simulink model "PTB_BatteryElectricVehicles"  (R2018b)
settings: Solver=ode23tb  StartTime=0.0  StopTime=3158  FixedStep=.001  RelTol=1e-5
model workspace (MAT data in the model file):
  Cd = 0.3
  DrCycles : struct (value not decoded)
  DriveCycleTime = 3158
  MCOS : class17 (value not decoded)
  I = 1
  Kbr = 5000
  P = 200
  axle_b = 10
  axle_k = 0.3
  bevAxle_wc = 400
  bevNp = 1
  bevNs = 8
  diffRatio = 1
  diffRatio1 = 1
  motorMaxTorqueNm = [0.6 0.6 0.8 0.9 2.2 2.9 5.1 7.8 11.3 15.3 20 25 ... (40 elements, 40x1)]
  motorSpeedRadPs = [90.118 90.118 90.118 90.118 90.01333333 89.804 89.49 89.07133333 88.65266667 88.12933333 87.39666667 86.87333333 ... (39 elements, 39x1)]
  vehicleMass = 365
  wheelRadius = 0.3
undefined symbols (not defined in the file): Driver, Wheels_Driver_VehDyn_Lib
libraries: autolibshared x3, simulink x2, autolibdatasheetbattery x1, autolibmappedmotor x1
(part 3 of 3)

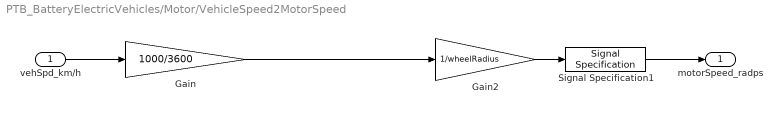
== system PTB_BatteryElectricVehicles/Motor/VehicleSpeed2MotorSpeed ==
  vehSpd_km/h : Inport
  Gain : Gain  Gain=1000/3600
  Gain2 : Gain  Gain=1/wheelRadius
  Signal Specification1 : SignalSpecification  Unit=rad/s
  motorSpeed_radps : Outport
  wires:
  Signal Specification1/1 -> motorSpeed_radps/1
  Gain/1 -> Gain2/1
  Gain2/1 -> Signal Specification1/1
  vehSpd_km/h/1 -> Gain/1
